simulink model "final_2_wo_capacitor"  (R2020b)
settings: Solver=VariableStepAuto  StartTime=0.0  StopTime=10  RelTol=1e-3
libraries: powerlib x23, powerlib_meascontrol x1
settings Model: Creator=SB Shuvo  LastModifiedBy=SB Shuvo
settings SolverCC: AlgebraicLoopSolver=LineSearch

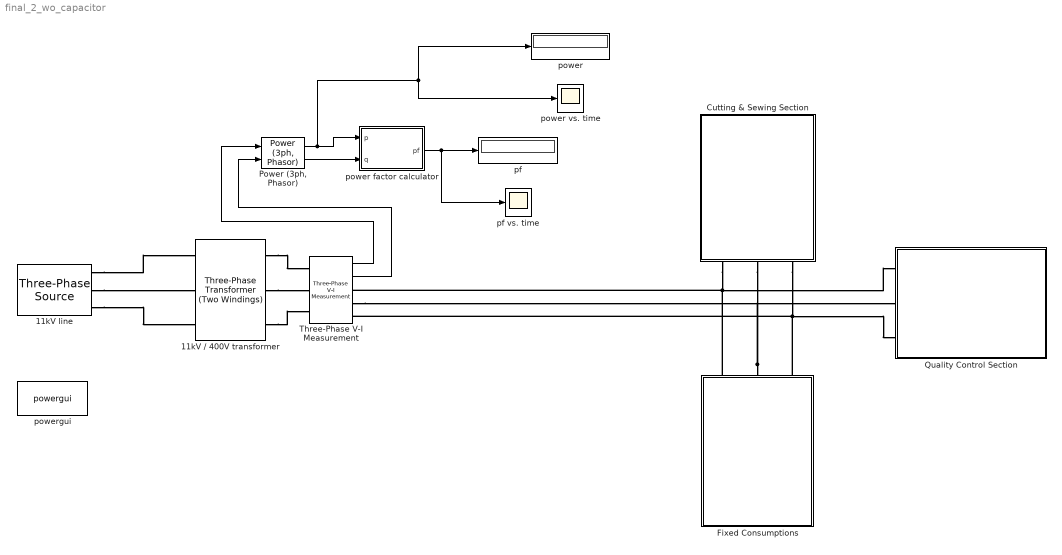
== system final_2_wo_capacitor ==
  11kV / 400V transformer : powerlib/Elements/Three-Phase Transformer (Two Windings)  Winding1Connection=Yg  Winding2Connection=Yg  CoreType=Three single-phase transformers  SetSaturation=off  Hysteresis=off  DataFile='hysteresis'  SetInitialFlux=off  Measurements=None  UNITS=SI  NominalPower=[ 80e3 , 50 ]  Winding1=[11000 1e-6 1e-6]  Winding2=[400 1e-6 1e-6]  Rm=1e6  Lm=1e6  L0=0.5  Saturation=[0 0;0.66652 1910.3;277.72 2419.7]  InitialFluxes=[ 0.8 , -0.8 , 0.7 ]  BreakLoop=off  DiscreteSolver=Trapezoidal iterative  DataType=on  TransfoNumber=1
  11kV line : powerlib/Electrical Sources/Three-Phase Source  InternalConnection=Yg  VoltagePhases=off  Voltage=11e3  PhaseAngle=0  Voltage_phases=[25e3 25e3 25e3]/sqrt(3)  PhaseAngles_phases=[0 -120 +120]  Frequency=50  NonIdealSource=on  SpecifyImpedance=off  Resistance=0.8929  Inductance=16.58e-3  ShortCircuitLevel=100e6  BaseVoltage=25e3  XRratio=7  BusType=swing  Pref=10e3  Qref=0  Prefabc=[10e3, 10e3, 10e3]  Qrefabc=[0, 0, 0]  Qmin=-inf  Qmax=inf
  Cutting & Sewing Section : Subsystem
  Fixed Consumptions : Subsystem
  "Power (3ph, Phasor)" : powerlib_meascontrol/Measurements/Power (3ph, Phasor)
      settings: SourceProductBaseCode=PS
  Quality Control Section : Subsystem
  Three-Phase V-I Measurement : powerlib/Measurements/Three-Phase V-I Measurement  VoltageMeasurement=phase-to-ground  SetLabelV=off  LabelV=Vabc  Vpu=off  VpuLL=off  CurrentMeasurement=yes  SetLabelI=off  LabelI=Iabc  Ipu=off  Pbase=100e6  Vbase=500e3  OutputType=Complex  PhasorSimulation=on  PSBequivalent=0
  pf : Display
  pf vs. time : Scope
  power : Display
  power factor calculator : MATLAB Function  TreatAsAtomicUnit=on
  power vs. time : Scope
  powergui : powerlib/powergui  Priority=1  SimulationMode=Phasor  SampleTime=50e-6  frequency=50  Iterations=50  frequencyindice=50  Pbase=100e6  ErrMax=1e-4  UnitsV=kV  UnitsW=MW  buscounter=2  FunctionMessages=off  echomessages=off  EnableUseOfTLC=off  CurrentSourceSwitches=off  DisableSnubberDevices=off  DisableRonSwitches=off  DisableVfSwitches=off  DisplayEquations=off  AutomaticDiscreteSolvers=off  SolverType=Tustin/Backward Euler (TBE)  Interpol=off  ExternalGateDelay=off  methode=off  Ts=100  x0status=blocks  SPID=on  SwTol=0  HookPort=off  NonlinearTolerance=1e-4  nMaxIteration=100  ContinueOnMaxIteration=off  RestoreLinks=warning  ResistiveCurrentMeasurement=off  Frange=[0:2:500]  Ylog=off  Xlog=on  ShowGrid=off  save=off  variable=ZData  structure=0  ZoomFFT=off  StartTime=0.0  cycles=1  DisplayStyle=1  fundamental=60  FreqAxis=off  MaxFrequency=1000  frequencyindicesteady=1  RmsSteady=1  display=off
  wires:
  "Power (3ph, Phasor)"/1 -> power vs. time/1, power/1, power factor calculator/1(p)
  "Power (3ph, Phasor)"/2 -> power factor calculator/2(q)
  power factor calculator/1(pf) -> pf vs. time/1, pf/1
  Three-Phase V-I Measurement/2 -> "Power (3ph, Phasor)"/2
  Three-Phase V-I Measurement/1 -> "Power (3ph, Phasor)"/1
  connections:
  11kV line/RConn1 -- 11kV / 400V transformer/LConn1
  11kV line/RConn2 -- 11kV / 400V transformer/LConn2
  11kV line/RConn3 -- 11kV / 400V transformer/LConn3
  11kV / 400V transformer/RConn3 -- Three-Phase V-I Measurement/LConn3
  11kV / 400V transformer/RConn2 -- Three-Phase V-I Measurement/LConn2
  11kV / 400V transformer/RConn1 -- Three-Phase V-I Measurement/LConn1
  Fixed Consumptions/LConn3 -- Quality Control Section/LConn3 -- Cutting & Sewing Section/LConn3 -- Three-Phase V-I Measurement/RConn3
  Cutting & Sewing Section/LConn1 -- Three-Phase V-I Measurement/RConn1 -- Quality Control Section/LConn1 -- Fixed Consumptions/LConn1
  Fixed Consumptions/LConn2 -- Three-Phase V-I Measurement/RConn2 -- Cutting & Sewing Section/LConn2 -- Quality Control Section/LConn2

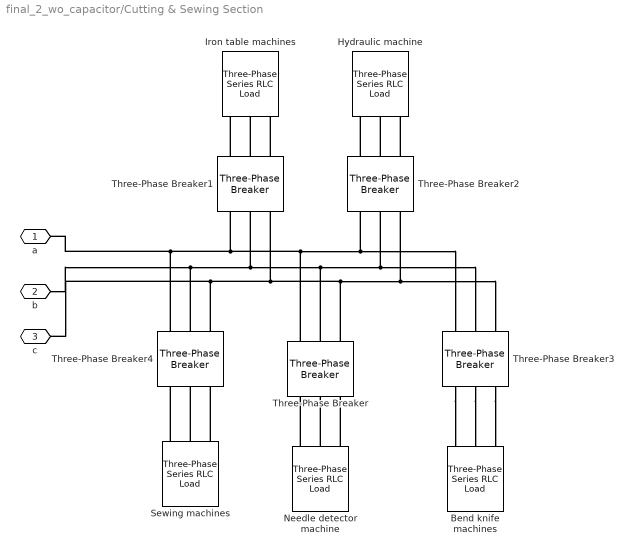
== system final_2_wo_capacitor/Cutting & Sewing Section ==
  Bend knife machines : powerlib/Elements/Three-Phase Series RLC Load  LConnTagsString=A|B|C  Configuration=Y (grounded)  NominalVoltage=400  Vabc=[1e3 1e3 1e3]  Vabcp=[1e3 1e3 1e3]  NominalFrequency=50  UnbalancedPower=off  ActivePower=3360  InductivePower=1500  CapacitivePower=0  Pabc=[10e3 9e3 11e3]  QLabc=[100 90 110]  QCabc=[100 90 110]  Pabcp=[10e3 9e3 11e3]  QLabcp=[100 90 110]  QCabcp=[100 90 110]  Measurements=None  LoadType=constant Z
  Hydraulic machine : powerlib/Elements/Three-Phase Series RLC Load  LConnTagsString=A|B|C  Configuration=Y (grounded)  NominalVoltage=400  Vabc=[1e3 1e3 1e3]  Vabcp=[1e3 1e3 1e3]  NominalFrequency=50  UnbalancedPower=off  ActivePower=2e3  InductivePower=1000  CapacitivePower=0  Pabc=[10e3 9e3 11e3]  QLabc=[100 90 110]  QCabc=[100 90 110]  Pabcp=[10e3 9e3 11e3]  QLabcp=[100 90 110]  QCabcp=[100 90 110]  Measurements=None  LoadType=constant Z
  Iron table machines : powerlib/Elements/Three-Phase Series RLC Load  LConnTagsString=A|B|C  Configuration=Y (grounded)  NominalVoltage=400  Vabc=[1e3 1e3 1e3]  Vabcp=[1e3 1e3 1e3]  NominalFrequency=50  UnbalancedPower=off  ActivePower=33e3  InductivePower=20e3  CapacitivePower=0  Pabc=[10e3 9e3 11e3]  QLabc=[100 90 110]  QCabc=[100 90 110]  Pabcp=[10e3 9e3 11e3]  QLabcp=[100 90 110]  QCabcp=[100 90 110]  Measurements=None  LoadType=constant Z
  Needle detector machine : powerlib/Elements/Three-Phase Series RLC Load  LConnTagsString=A|B|C  Configuration=Y (grounded)  NominalVoltage=400  Vabc=[1e3 1e3 1e3]  Vabcp=[1e3 1e3 1e3]  NominalFrequency=50  UnbalancedPower=off  ActivePower=150  InductivePower=100  CapacitivePower=0  Pabc=[10e3 9e3 11e3]  QLabc=[100 90 110]  QCabc=[100 90 110]  Pabcp=[10e3 9e3 11e3]  QLabcp=[100 90 110]  QCabcp=[100 90 110]  Measurements=None  LoadType=constant Z
  Sewing machines : powerlib/Elements/Three-Phase Series RLC Load  LConnTagsString=A|B|C  Configuration=Y (grounded)  NominalVoltage=400  Vabc=[1e3 1e3 1e3]  Vabcp=[1e3 1e3 1e3]  NominalFrequency=50  UnbalancedPower=off  ActivePower=9000  InductivePower=4e3  CapacitivePower=0  Pabc=[10e3 9e3 11e3]  QLabc=[100 90 110]  QCabc=[100 90 110]  Pabcp=[10e3 9e3 11e3]  QLabcp=[100 90 110]  QCabcp=[100 90 110]  Measurements=None  LoadType=constant Z
  Three-Phase Breaker : powerlib/Elements/Three-Phase Breaker  InitialState=open  SwitchA=on  SwitchB=on  SwitchC=on  SwitchTimes=[0.5 5 6]  External=off  BreakerResistance=0.01  SnubberResistance=1e6  SnubberCapacitance=inf  Measurements=None
  Three-Phase Breaker1 : powerlib/Elements/Three-Phase Breaker  InitialState=open  SwitchA=on  SwitchB=on  SwitchC=on  SwitchTimes=[0.5 5 6]  External=off  BreakerResistance=0.01  SnubberResistance=1e6  SnubberCapacitance=inf  Measurements=None
  Three-Phase Breaker2 : powerlib/Elements/Three-Phase Breaker  InitialState=open  SwitchA=on  SwitchB=on  SwitchC=on  SwitchTimes=[0.5 5 6 8]  External=off  BreakerResistance=0.01  SnubberResistance=1e6  SnubberCapacitance=inf  Measurements=None
  Three-Phase Breaker3 : powerlib/Elements/Three-Phase Breaker  InitialState=open  SwitchA=on  SwitchB=on  SwitchC=on  SwitchTimes=[0.5 5 6 8]  External=off  BreakerResistance=0.01  SnubberResistance=1e6  SnubberCapacitance=inf  Measurements=None
  Three-Phase Breaker4 : powerlib/Elements/Three-Phase Breaker  InitialState=open  SwitchA=on  SwitchB=on  SwitchC=on  SwitchTimes=[0.5 5 6]  External=off  BreakerResistance=0.01  SnubberResistance=1e6  SnubberCapacitance=inf  Measurements=None
  a : PMIOPort  Side=Left
  b : PMIOPort  Port=2  Side=Left
  c : PMIOPort  Port=3  Side=Left
  connections:
  Three-Phase Breaker2/LConn2 -- Three-Phase Breaker3/RConn2 -- Three-Phase Breaker4/RConn2 -- b/RConn1 -- Three-Phase Breaker1/LConn2 -- Three-Phase Breaker/RConn2
  Sewing machines/LConn3 -- Three-Phase Breaker4/LConn3
  Sewing machines/LConn1 -- Three-Phase Breaker4/LConn1
  Needle detector machine/LConn2 -- Three-Phase Breaker/LConn2
  Needle detector machine/LConn3 -- Three-Phase Breaker/LConn3
  Needle detector machine/LConn1 -- Three-Phase Breaker/LConn1
  Three-Phase Breaker1/RConn1 -- Iron table machines/LConn1
  Three-Phase Breaker1/RConn3 -- Iron table machines/LConn3
  Three-Phase Breaker1/RConn2 -- Iron table machines/LConn2
  Three-Phase Breaker2/RConn1 -- Hydraulic machine/LConn1
  Three-Phase Breaker2/RConn2 -- Hydraulic machine/LConn2
  Three-Phase Breaker2/RConn3 -- Hydraulic machine/LConn3
  Three-Phase Breaker3/LConn2 -- Bend knife machines/LConn2
  Three-Phase Breaker3/LConn3 -- Bend knife machines/LConn3
  Three-Phase Breaker3/LConn1 -- Bend knife machines/LConn1
  Three-Phase Breaker/RConn1 -- Three-Phase Breaker1/LConn1 -- Three-Phase Breaker4/RConn1 -- a/RConn1 -- Three-Phase Breaker3/RConn1 -- Three-Phase Breaker2/LConn1
  Three-Phase Breaker/RConn3 -- Three-Phase Breaker1/LConn3 -- Three-Phase Breaker4/RConn3 -- c/RConn1 -- Three-Phase Breaker3/RConn3 -- Three-Phase Breaker2/LConn3
  Sewing machines/LConn2 -- Three-Phase Breaker4/LConn2

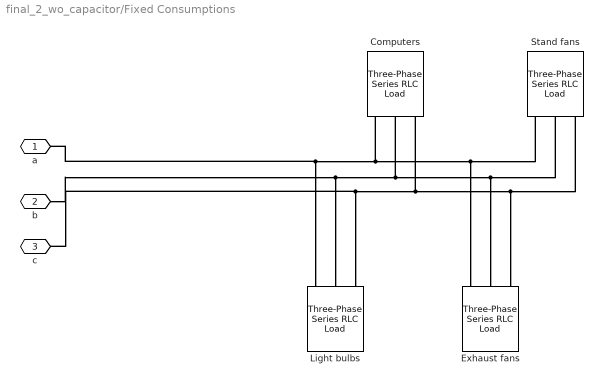
== system final_2_wo_capacitor/Fixed Consumptions ==
  Computers : powerlib/Elements/Three-Phase Series RLC Load  LConnTagsString=A|B|C  Configuration=Y (grounded)  NominalVoltage=400  Vabc=[1e3 1e3 1e3]  Vabcp=[1e3 1e3 1e3]  NominalFrequency=50  UnbalancedPower=off  ActivePower=5e3  InductivePower=200  CapacitivePower=100  Pabc=[10e3 9e3 11e3]  QLabc=[100 90 110]  QCabc=[100 90 110]  Pabcp=[10e3 9e3 11e3]  QLabcp=[100 90 110]  QCabcp=[100 90 110]  Measurements=None  LoadType=constant Z
  Exhaust fans : powerlib/Elements/Three-Phase Series RLC Load  LConnTagsString=A|B|C  Configuration=Y (grounded)  NominalVoltage=400  Vabc=[1e3 1e3 1e3]  Vabcp=[1e3 1e3 1e3]  NominalFrequency=50  UnbalancedPower=off  ActivePower=2100  InductivePower=1000  CapacitivePower=0  Pabc=[10e3 9e3 11e3]  QLabc=[100 90 110]  QCabc=[100 90 110]  Pabcp=[10e3 9e3 11e3]  QLabcp=[100 90 110]  QCabcp=[100 90 110]  Measurements=None  LoadType=constant Z
  Light bulbs : powerlib/Elements/Three-Phase Series RLC Load  LConnTagsString=A|B|C  Configuration=Y (grounded)  NominalVoltage=400  Vabc=[1e3 1e3 1e3]  Vabcp=[1e3 1e3 1e3]  NominalFrequency=50  UnbalancedPower=off  ActivePower=3e3  InductivePower=0  CapacitivePower=0  Pabc=[10e3 9e3 11e3]  QLabc=[100 90 110]  QCabc=[100 90 110]  Pabcp=[10e3 9e3 11e3]  QLabcp=[100 90 110]  QCabcp=[100 90 110]  Measurements=None  LoadType=constant Z
  Stand fans : powerlib/Elements/Three-Phase Series RLC Load  LConnTagsString=A|B|C  Configuration=Y (grounded)  NominalVoltage=400  Vabc=[1e3 1e3 1e3]  Vabcp=[1e3 1e3 1e3]  NominalFrequency=50  UnbalancedPower=off  ActivePower=1050  InductivePower=400  CapacitivePower=0  Pabc=[10e3 9e3 11e3]  QLabc=[100 90 110]  QCabc=[100 90 110]  Pabcp=[10e3 9e3 11e3]  QLabcp=[100 90 110]  QCabcp=[100 90 110]  Measurements=None  LoadType=constant Z
  a : PMIOPort  Side=Left
  b : PMIOPort  Port=2  Side=Left
  c : PMIOPort  Port=3  Side=Left
  connections:
  a/RConn1 -- Light bulbs/LConn1 -- Exhaust fans/LConn1 -- Stand fans/LConn1 -- Computers/LConn1
  Light bulbs/LConn3 -- c/RConn1 -- Stand fans/LConn3 -- Exhaust fans/LConn3 -- Computers/LConn3
  b/RConn1 -- Light bulbs/LConn2 -- Exhaust fans/LConn2 -- Stand fans/LConn2 -- Computers/LConn2

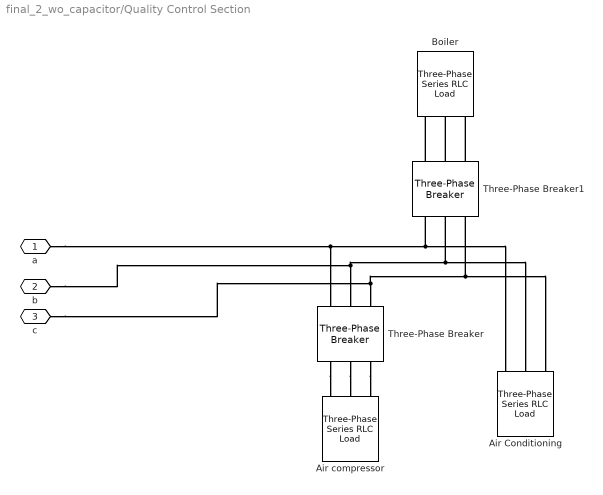
== system final_2_wo_capacitor/Quality Control Section ==
  Air Conditioning : powerlib/Elements/Three-Phase Series RLC Load  LConnTagsString=A|B|C  Configuration=Y (grounded)  NominalVoltage=400  Vabc=[1e3 1e3 1e3]  Vabcp=[1e3 1e3 1e3]  NominalFrequency=50  UnbalancedPower=off  ActivePower=610  InductivePower=300  CapacitivePower=0  Pabc=[10e3 9e3 11e3]  QLabc=[100 90 110]  QCabc=[100 90 110]  Pabcp=[10e3 9e3 11e3]  QLabcp=[100 90 110]  QCabcp=[100 90 110]  Measurements=None  LoadType=constant Z
  Air compressor : powerlib/Elements/Three-Phase Series RLC Load  LConnTagsString=A|B|C  Configuration=Y (grounded)  NominalVoltage=400  Vabc=[1e3 1e3 1e3]  Vabcp=[1e3 1e3 1e3]  NominalFrequency=50  UnbalancedPower=off  ActivePower=11e3  InductivePower=5e3  CapacitivePower=0  Pabc=[10e3 9e3 11e3]  QLabc=[100 90 110]  QCabc=[100 90 110]  Pabcp=[10e3 9e3 11e3]  QLabcp=[100 90 110]  QCabcp=[100 90 110]  Measurements=None  LoadType=constant Z
  Boiler : powerlib/Elements/Three-Phase Series RLC Load  LConnTagsString=A|B|C  Configuration=Y (grounded)  NominalVoltage=400  Vabc=[1e3 1e3 1e3]  Vabcp=[1e3 1e3 1e3]  NominalFrequency=50  UnbalancedPower=off  ActivePower=536  InductivePower=250  CapacitivePower=0  Pabc=[10e3 9e3 11e3]  QLabc=[100 90 110]  QCabc=[100 90 110]  Pabcp=[10e3 9e3 11e3]  QLabcp=[100 90 110]  QCabcp=[100 90 110]  Measurements=None  LoadType=constant Z
  Three-Phase Breaker : powerlib/Elements/Three-Phase Breaker  InitialState=open  SwitchA=on  SwitchB=on  SwitchC=on  SwitchTimes=[0.5 5 6 9]  External=off  BreakerResistance=0.01  SnubberResistance=1e6  SnubberCapacitance=inf  Measurements=None
  Three-Phase Breaker1 : powerlib/Elements/Three-Phase Breaker  InitialState=open  SwitchA=on  SwitchB=on  SwitchC=on  SwitchTimes=[0.5 5 6 8]  External=off  BreakerResistance=0.01  SnubberResistance=1e6  SnubberCapacitance=inf  Measurements=None
  a : PMIOPort  Side=Left
  b : PMIOPort  Port=2  Side=Left
  c : PMIOPort  Port=3  Side=Left
  connections:
  Three-Phase Breaker1/RConn1 -- Boiler/LConn1
  c/RConn1 -- Air Conditioning/LConn3 -- Three-Phase Breaker1/LConn3 -- Three-Phase Breaker/RConn3
  b/RConn1 -- Air Conditioning/LConn2 -- Three-Phase Breaker1/LConn2 -- Three-Phase Breaker/RConn2
  Three-Phase Breaker/LConn2 -- Air compressor/LConn2
  Three-Phase Breaker/LConn3 -- Air compressor/LConn3
  Three-Phase Breaker/LConn1 -- Air compressor/LConn1
  a/RConn1 -- Air Conditioning/LConn1 -- Three-Phase Breaker1/LConn1 -- Three-Phase Breaker/RConn1
  Three-Phase Breaker1/RConn3 -- Boiler/LConn3
  Three-Phase Breaker1/RConn2 -- Boiler/LConn2

== matlab function final_2_wo_capacitor/power factor calculator ==
  data: p input; pf output; q input
function pf = fcn(p,q)

pf = p/sqrt(p^2 + q^2);
